simulink model "HybridBus_PerformanceModel"  (R2025a)
settings: Solver=VariableStepAuto  StartTime=0.0  StopTime=10.0  RelTol=1e-3
undefined symbols (not defined in the file): air_density_kg_m3, DiscIntNeverNeededParam, drag_coefficient, final_drive_motoring_efficiency, frontal_area_m2, gravity_m_s2, model_sample_time_s, motor_peak_power_kw, performance_battery_available_power_kw, performance_driver_kp_s, performance_low_speed_protection_m_s, performance_max_acceleration_m_s2, performance_max_deceleration_m_s2, performance_motor_wheel_force_limit_n, performance_route_aux_multiplier, performance_route_distance_m, performance_route_grade_pct, performance_route_speed_m_s, rolling_coefficient, vehicle_mass_kg
libraries: simulink x4
settings Model: Creator=Karuna  LastModifiedBy=Karuna

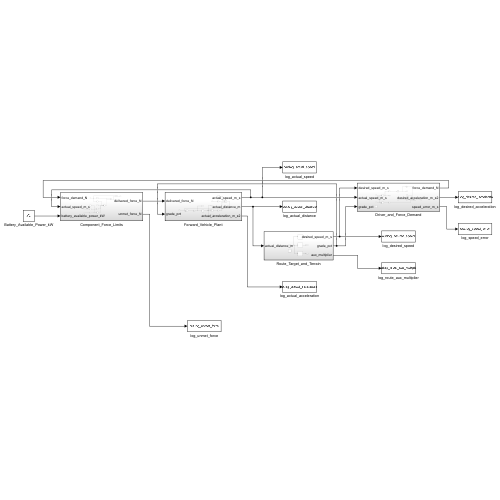
[thumbnail: Simulink's stored preview of the top-level diagram]
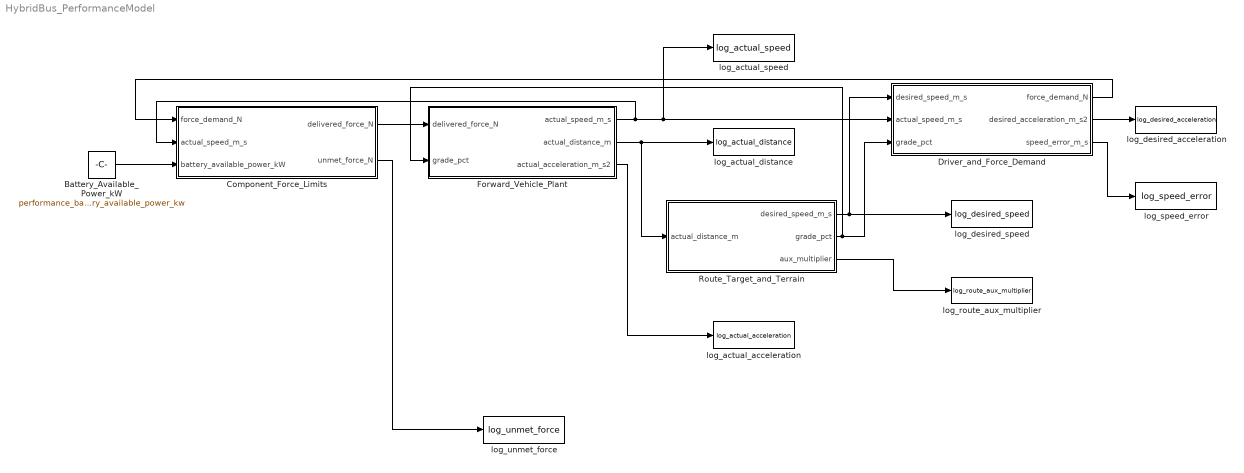
== system HybridBus_PerformanceModel ==
  Battery_Available_Power_kW : Constant  Value=performance_battery_available_power_kw
  Component_Force_Limits : Subsystem
  Driver_and_Force_Demand : Subsystem
  Forward_Vehicle_Plant : Subsystem
  Route_Target_and_Terrain : Subsystem
  log_actual_acceleration : ToWorkspace  VariableName=log_actual_acceleration  SaveFormat=Timeseries  SampleTime=-1
  log_actual_distance : ToWorkspace  VariableName=log_actual_distance  SaveFormat=Timeseries  SampleTime=-1
  log_actual_speed : ToWorkspace  VariableName=log_actual_speed  SaveFormat=Timeseries  SampleTime=-1
  log_desired_acceleration : ToWorkspace  VariableName=log_desired_acceleration  SaveFormat=Timeseries  SampleTime=-1
  log_desired_speed : ToWorkspace  VariableName=log_desired_speed  SaveFormat=Timeseries  SampleTime=-1
  log_route_aux_multiplier : ToWorkspace  VariableName=log_route_aux_multiplier  SaveFormat=Timeseries  SampleTime=-1
  log_speed_error : ToWorkspace  VariableName=log_speed_error  SaveFormat=Timeseries  SampleTime=-1
  log_unmet_force : ToWorkspace  VariableName=log_unmet_force  SaveFormat=Timeseries  SampleTime=-1
  wires:
  Route_Target_and_Terrain/3(aux_multiplier) -> log_route_aux_multiplier/1
  Forward_Vehicle_Plant/3(actual_acceleration_m_s2) -> log_actual_acceleration/1
  Driver_and_Force_Demand/2(desired_acceleration_m_s2) -> log_desired_acceleration/1
  Forward_Vehicle_Plant/2(actual_distance_m) -> Route_Target_and_Terrain/1(actual_distance_m), log_actual_distance/1
  Route_Target_and_Terrain/1(desired_speed_m_s) -> log_desired_speed/1, Driver_and_Force_Demand/1(desired_speed_m_s)
  Forward_Vehicle_Plant/1(actual_speed_m_s) -> log_actual_speed/1, Driver_and_Force_Demand/2(actual_speed_m_s), Component_Force_Limits/2(actual_speed_m_s)
  Route_Target_and_Terrain/2(grade_pct) -> Forward_Vehicle_Plant/2(grade_pct), Driver_and_Force_Demand/3(grade_pct)
  Driver_and_Force_Demand/1(force_demand_N) -> Component_Force_Limits/1(force_demand_N)
  Battery_Available_Power_kW/1 -> Component_Force_Limits/3(battery_available_power_kW)
  Component_Force_Limits/1(delivered_force_N) -> Forward_Vehicle_Plant/1(delivered_force_N)
  Driver_and_Force_Demand/3(speed_error_m_s) -> log_speed_error/1
  Component_Force_Limits/2(unmet_force_N) -> log_unmet_force/1

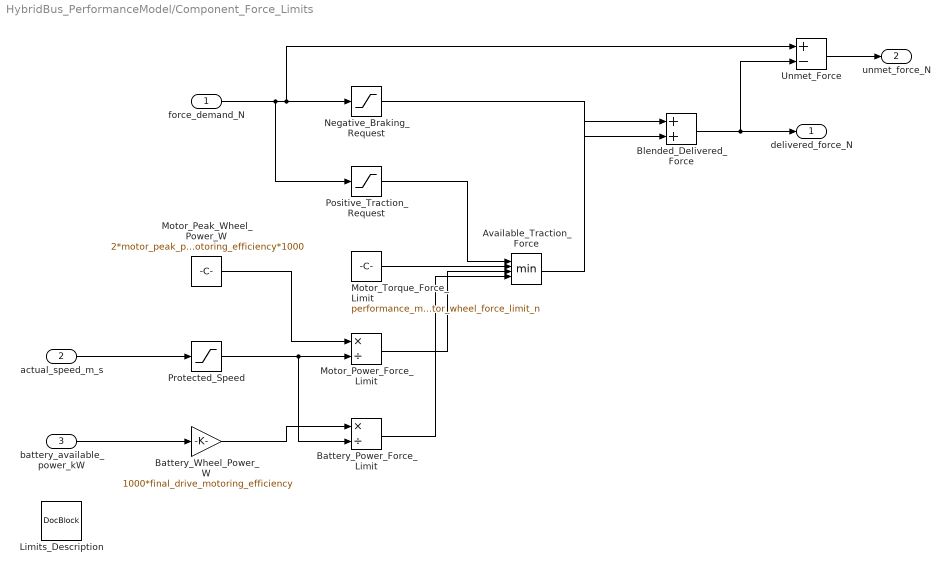
== system HybridBus_PerformanceModel/Component_Force_Limits ==
  force_demand_N : Inport
  actual_speed_m_s : Inport  Port=2
  battery_available_power_kW : Inport  Port=3
  Available_Traction_Force : MinMax  Inputs=4
  Battery_Power_Force_Limit : Product  Inputs=*/
  Battery_Wheel_Power_W : Gain  Gain=1000*final_drive_motoring_efficiency
  Blended_Delivered_Force : Sum
  Limits_Description : simulink/Model-Wide Utilities/DocBlock  Description=Positive force is limited by motor torque, motor power, and available battery DC power. Negative force uses ideal blended regeneration and pneumatic braking in this plant-level model.  DocumentType=Text
      settings: LibrarySourceBlock=|
      | hdlsllib/Model-Wide
      | Utilities/DocBlock
  Motor_Peak_Wheel_Power_W : Constant  Value=2*motor_peak_power_kw*final_drive_motoring_efficiency*1000
  Motor_Power_Force_Limit : Product  Inputs=*/
  Motor_Torque_Force_Limit : Constant  Value=performance_motor_wheel_force_limit_n
  Negative_Braking_Request : Saturate  UpperLimit=0  LowerLimit=-inf
  Positive_Traction_Request : Saturate  UpperLimit=inf  LowerLimit=0
  Protected_Speed : Saturate  UpperLimit=inf  LowerLimit=performance_low_speed_protection_m_s
  Unmet_Force : Sum  Inputs=+-
  delivered_force_N : Outport
  unmet_force_N : Outport  Port=2
  wires:
  force_demand_N/1 -> Unmet_Force/1, Negative_Braking_Request/1, Positive_Traction_Request/1
  actual_speed_m_s/1 -> Protected_Speed/1
  Motor_Peak_Wheel_Power_W/1 -> Motor_Power_Force_Limit/1
  Protected_Speed/1 -> Battery_Power_Force_Limit/2, Motor_Power_Force_Limit/2
  battery_available_power_kW/1 -> Battery_Wheel_Power_W/1
  Battery_Wheel_Power_W/1 -> Battery_Power_Force_Limit/1
  Positive_Traction_Request/1 -> Available_Traction_Force/1
  Motor_Torque_Force_Limit/1 -> Available_Traction_Force/2
  Motor_Power_Force_Limit/1 -> Available_Traction_Force/3
  Battery_Power_Force_Limit/1 -> Available_Traction_Force/4
  Available_Traction_Force/1 -> Blended_Delivered_Force/1
  Negative_Braking_Request/1 -> Blended_Delivered_Force/2
  Blended_Delivered_Force/1 -> delivered_force_N/1, Unmet_Force/2
  Unmet_Force/1 -> unmet_force_N/1

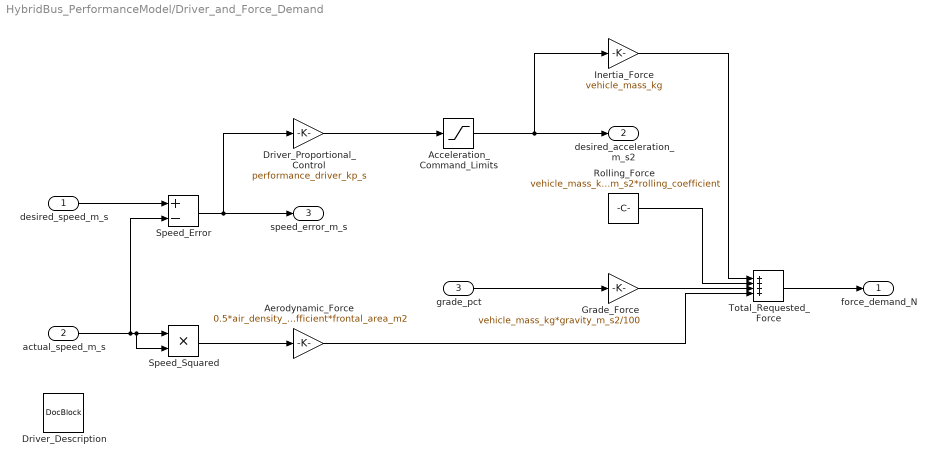
== system HybridBus_PerformanceModel/Driver_and_Force_Demand ==
  desired_speed_m_s : Inport
  actual_speed_m_s : Inport  Port=2
  grade_pct : Inport  Port=3
  Acceleration_Command_Limits : Saturate  UpperLimit=performance_max_acceleration_m_s2  LowerLimit=-performance_max_deceleration_m_s2
  Aerodynamic_Force : Gain  Gain=0.5*air_density_kg_m3*drag_coefficient*frontal_area_m2
  Driver_Description : simulink/Model-Wide Utilities/DocBlock  Description=The driver converts desired-minus-actual speed into a bounded acceleration request. Inertia, rolling, grade, and aerodynamic forces form the demanded wheel force.  DocumentType=Text
      settings: LibrarySourceBlock=|
      | hdlsllib/Model-Wide
      | Utilities/DocBlock
  Driver_Proportional_Control : Gain  Gain=performance_driver_kp_s
  Grade_Force : Gain  Gain=vehicle_mass_kg*gravity_m_s2/100
  Inertia_Force : Gain  Gain=vehicle_mass_kg
  Rolling_Force : Constant  Value=vehicle_mass_kg*gravity_m_s2*rolling_coefficient
  Speed_Error : Sum  Inputs=+-
  Speed_Squared : Product  Inputs=**
  Total_Requested_Force : Sum  Inputs=++++
  force_demand_N : Outport
  desired_acceleration_m_s2 : Outport  Port=2
  speed_error_m_s : Outport  Port=3
  wires:
  desired_speed_m_s/1 -> Speed_Error/1
  actual_speed_m_s/1 -> Speed_Squared/2, Speed_Squared/1, Speed_Error/2
  Speed_Error/1 -> speed_error_m_s/1, Driver_Proportional_Control/1
  Driver_Proportional_Control/1 -> Acceleration_Command_Limits/1
  Acceleration_Command_Limits/1 -> desired_acceleration_m_s2/1, Inertia_Force/1
  grade_pct/1 -> Grade_Force/1
  Speed_Squared/1 -> Aerodynamic_Force/1
  Inertia_Force/1 -> Total_Requested_Force/1
  Rolling_Force/1 -> Total_Requested_Force/2
  Grade_Force/1 -> Total_Requested_Force/3
  Aerodynamic_Force/1 -> Total_Requested_Force/4
  Total_Requested_Force/1 -> force_demand_N/1

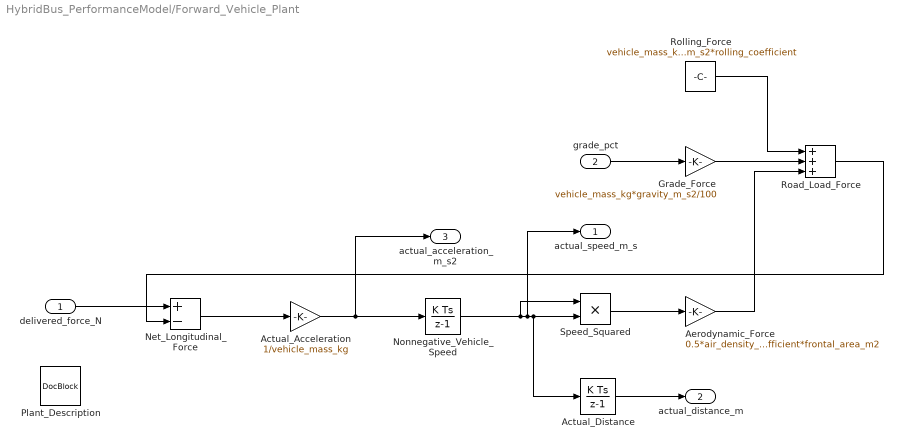
== system HybridBus_PerformanceModel/Forward_Vehicle_Plant ==
  delivered_force_N : Inport
  grade_pct : Inport  Port=2
  Actual_Acceleration : Gain  Gain=1/vehicle_mass_kg
  Actual_Distance : DiscreteIntegrator  SampleTime=model_sample_time_s  ICPrevOutput=DiscIntNeverNeededParam  ICPrevScaledInput=DiscIntNeverNeededParam
  Aerodynamic_Force : Gain  Gain=0.5*air_density_kg_m3*drag_coefficient*frontal_area_m2
  Grade_Force : Gain  Gain=vehicle_mass_kg*gravity_m_s2/100
  Net_Longitudinal_Force : Sum  Inputs=+-
  Nonnegative_Vehicle_Speed : DiscreteIntegrator  SampleTime=model_sample_time_s  LimitOutput=on  LowerSaturationLimit=0  ICPrevOutput=DiscIntNeverNeededParam  ICPrevScaledInput=DiscIntNeverNeededParam
  Plant_Description : simulink/Model-Wide Utilities/DocBlock  Description=Delivered wheel force minus rolling, grade, and aerodynamic road loads determines actual acceleration. Speed is integrated with a zero lower bound to prevent rollback; actual speed integrates to travelled distance.  DocumentType=Text
      settings: LibrarySourceBlock=|
      | hdlsllib/Model-Wide
      | Utilities/DocBlock
  Road_Load_Force : Sum  Inputs=+++
  Rolling_Force : Constant  Value=vehicle_mass_kg*gravity_m_s2*rolling_coefficient
  Speed_Squared : Product  Inputs=**
  actual_speed_m_s : Outport
  actual_distance_m : Outport  Port=2
  actual_acceleration_m_s2 : Outport  Port=3
  wires:
  Actual_Distance/1 -> actual_distance_m/1
  Actual_Acceleration/1 -> Nonnegative_Vehicle_Speed/1, actual_acceleration_m_s2/1
  Net_Longitudinal_Force/1 -> Actual_Acceleration/1
  Road_Load_Force/1 -> Net_Longitudinal_Force/2
  delivered_force_N/1 -> Net_Longitudinal_Force/1
  Aerodynamic_Force/1 -> Road_Load_Force/3
  Grade_Force/1 -> Road_Load_Force/2
  Rolling_Force/1 -> Road_Load_Force/1
  Speed_Squared/1 -> Aerodynamic_Force/1
  Nonnegative_Vehicle_Speed/1 -> Actual_Distance/1, Speed_Squared/2, actual_speed_m_s/1, Speed_Squared/1
  grade_pct/1 -> Grade_Force/1

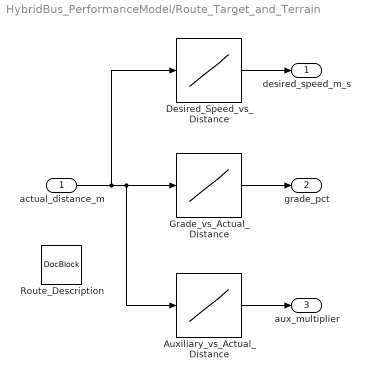
== system HybridBus_PerformanceModel/Route_Target_and_Terrain ==
  actual_distance_m : Inport
  Auxiliary_vs_Actual_Distance : Lookup_n-D  NumberOfTableDimensions=1  BreakpointsForDimension1=performance_route_distance_m  Table=performance_route_aux_multiplier  InternalRulePriority=Speed  RndMeth=Simplest
  Desired_Speed_vs_Distance : Lookup_n-D  NumberOfTableDimensions=1  BreakpointsForDimension1=performance_route_distance_m  Table=performance_route_speed_m_s  InternalRulePriority=Speed  RndMeth=Simplest
  Grade_vs_Actual_Distance : Lookup_n-D  NumberOfTableDimensions=1  BreakpointsForDimension1=performance_route_distance_m  Table=performance_route_grade_pct  InternalRulePriority=Speed  RndMeth=Simplest
  Route_Description : simulink/Model-Wide Utilities/DocBlock  Description=Route speed is a driver target. Grade and auxiliary multiplier are interpolated against actual travelled distance, so a delayed vehicle cannot skip terrain.  DocumentType=Text
      settings: LibrarySourceBlock=|
      | hdlsllib/Model-Wide
      | Utilities/DocBlock
  desired_speed_m_s : Outport
  grade_pct : Outport  Port=2
  aux_multiplier : Outport  Port=3
  wires:
  Auxiliary_vs_Actual_Distance/1 -> aux_multiplier/1
  Grade_vs_Actual_Distance/1 -> grade_pct/1
  Desired_Speed_vs_Distance/1 -> desired_speed_m_s/1
  actual_distance_m/1 -> Grade_vs_Actual_Distance/1, Auxiliary_vs_Actual_Distance/1, Desired_Speed_vs_Distance/1
